simulink model "Simulacion_con_vd_export"  (R2023b)
settings: Solver=VariableStepAuto  StartTime=0.0  StopTime=2.5  RelTol=1e-3
undefined symbols (not defined in the file): alpha_cu, b_eq, C_ts, id0, J_eq, k_l, L_d, L_ls, L_q, lambda_m, magnitude, P_p, r, R_sREF, R_ts_amb, T_amb, T_sREF
libraries: SignalEditorBlockLib x7
(part 1 of 2)
settings Model: Creator=tomas  LastModifiedBy=tomas

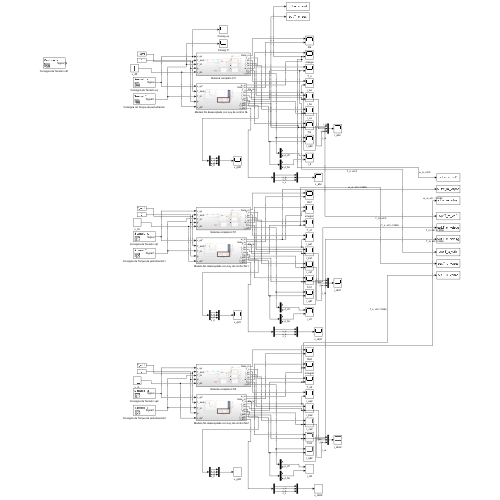
[thumbnail: Simulink's stored preview of the top-level diagram]
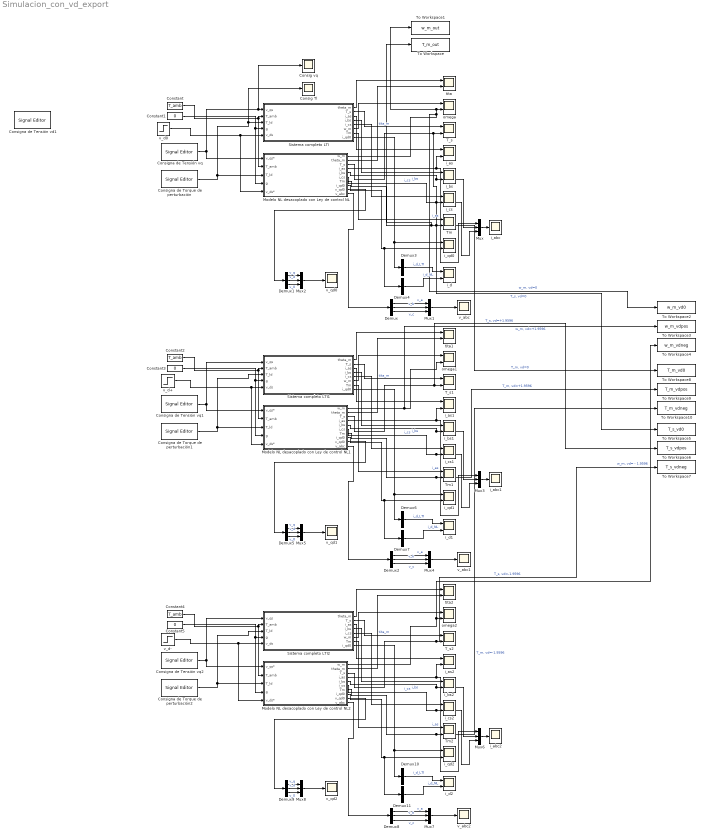
== system Simulacion_con_vd_export ==
  Consig Tl : Scope
  Consig vq : Scope
  Consigna de Tensión vd1 : SignalEditorBlockLib/Signal Editor  FileName=D:\Facu\Final AyME\Final-AyME\Simulink_LA\Simulacion\Señales\senial_vd.mat  ActiveScenario=Scenario_vd  ActiveSignal=Signal  IsBus=off  OutputBusObjectStr=Bus: BusObject  SampleTime=0  Interpolate=off  ZeroCross=off  OutputAfterFinalValue=Setting to zero  Unit=inherit  PreserveSignalName=on  ApplySigPropsToAllScenarios=on  ApplySigPropsToAllSignals=off
  Consigna de Tensión vq : SignalEditorBlockLib/Signal Editor  FileName=D:\Facu\Final AyME\Final-AyME\Simulink_LA\Simulacion\Señales\senial_vq.mat  ActiveScenario=Scenario_vq  ActiveSignal=Signal  IsBus=off  OutputBusObjectStr=Bus: BusObject  SampleTime=0  Interpolate=off  ZeroCross=off  OutputAfterFinalValue=Setting to zero  Unit=inherit  PreserveSignalName=on  ApplySigPropsToAllScenarios=on  ApplySigPropsToAllSignals=off
  Consigna de Tensión vq1 : SignalEditorBlockLib/Signal Editor  FileName=D:\Facu\Final AyME\Final-AyME\Simulink_LA\Simulacion\Señales\senial_vq.mat  ActiveScenario=Scenario_vq  ActiveSignal=Signal  IsBus=off  OutputBusObjectStr=Bus: BusObject  SampleTime=0  Interpolate=off  ZeroCross=off  OutputAfterFinalValue=Setting to zero  Unit=inherit  PreserveSignalName=on  ApplySigPropsToAllScenarios=on  ApplySigPropsToAllSignals=off
  Consigna de Tensión vq2 : SignalEditorBlockLib/Signal Editor  FileName=D:\Facu\Final AyME\Final-AyME\Simulink_LA\Simulacion\Señales\senial_vq.mat  ActiveScenario=Scenario_vq  ActiveSignal=Signal  IsBus=off  OutputBusObjectStr=Bus: BusObject  SampleTime=0  Interpolate=off  ZeroCross=off  OutputAfterFinalValue=Setting to zero  Unit=inherit  PreserveSignalName=on  ApplySigPropsToAllScenarios=on  ApplySigPropsToAllSignals=off
  Consigna de Torque de perturbación : SignalEditorBlockLib/Signal Editor  FileName=D:\Facu\Final AyME\Final-AyME\Simulink_LA\Simulacion\Señales\Signal_Tl.mat  ActiveScenario=ScenarioTl  ActiveSignal=Signal1  IsBus=off  OutputBusObjectStr=Bus: BusObject  SampleTime=0  Interpolate=off  ZeroCross=off  OutputAfterFinalValue=Setting to zero  Unit=inherit  PreserveSignalName=on  ApplySigPropsToAllScenarios=on  ApplySigPropsToAllSignals=off
  Consigna de Torque de perturbación1 : SignalEditorBlockLib/Signal Editor  FileName=D:\Facu\Final AyME\Final-AyME\Simulink_LA\Simulacion\Señales\Signal_Tl.mat  ActiveScenario=ScenarioTl  ActiveSignal=Signal1  IsBus=off  OutputBusObjectStr=Bus: BusObject  SampleTime=0  Interpolate=off  ZeroCross=off  OutputAfterFinalValue=Setting to zero  Unit=inherit  PreserveSignalName=on  ApplySigPropsToAllScenarios=on  ApplySigPropsToAllSignals=off
  Consigna de Torque de perturbación2 : SignalEditorBlockLib/Signal Editor  FileName=D:\Facu\Final AyME\Final-AyME\Simulink_LA\Simulacion\Señales\Signal_Tl.mat  ActiveScenario=ScenarioTl  ActiveSignal=Signal1  IsBus=off  OutputBusObjectStr=Bus: BusObject  SampleTime=0  Interpolate=off  ZeroCross=off  OutputAfterFinalValue=Setting to zero  Unit=inherit  PreserveSignalName=on  ApplySigPropsToAllScenarios=on  ApplySigPropsToAllSignals=off
  Constant : Constant  Value=T_amb
  Constant1 : Constant  Value=0
  Constant2 : Constant  Value=T_amb
  Constant3 : Constant  Value=0
  Constant4 : Constant  Value=T_amb
  Constant5 : Constant  Value=0
  Demux{,1..11} (12 alike) : Demux  Outputs=3
  Modelo NL desacoplado con Ley de control NL : Subsystem
  Modelo NL desacoplado con Ley de control NL1 : Subsystem
  Modelo NL desacoplado con Ley de control NL2 : Subsystem
  Mux{,1..8} (9 alike) : Mux  Inputs=3
  Sistema completo LTI : Subsystem
  Sistema completo LTI1 : Subsystem
  Sistema completo LTI2 : Subsystem
  T_s : Scope  NumInputPorts=2
  T_s1 : Scope  NumInputPorts=2
  T_s2 : Scope  NumInputPorts=2
  Tm : Scope  NumInputPorts=2
  Tm1 : Scope  NumInputPorts=2
  Tm2 : Scope  NumInputPorts=2
  To Workspace : ToWorkspace  VariableName=T_m_out  SampleTime=-1
  To Workspace1 : ToWorkspace  VariableName=w_m_out  SampleTime=-1
  To Workspace10 : ToWorkspace  VariableName=T_m_vdneg  SaveFormat=Structure With Time  SampleTime=-1
  To Workspace2 : ToWorkspace  VariableName=w_m_vd0  SaveFormat=Structure With Time  SampleTime=-1
  To Workspace3 : ToWorkspace  VariableName=w_m_vdpos  SaveFormat=Structure With Time  SampleTime=-1
  To Workspace4 : ToWorkspace  VariableName=w_m_vdneg  SaveFormat=Structure With Time  SampleTime=-1
  To Workspace5 : ToWorkspace  VariableName=T_s_vd0  SaveFormat=Structure With Time  SampleTime=-1
  To Workspace6 : ToWorkspace  VariableName=T_s_vdpos  SaveFormat=Structure With Time  SampleTime=-1
  To Workspace7 : ToWorkspace  VariableName=T_s_vdneg  SaveFormat=Structure With Time  SampleTime=-1
  To Workspace8 : ToWorkspace  VariableName=T_m_vd0  SaveFormat=Structure With Time  SampleTime=-1
  To Workspace9 : ToWorkspace  VariableName=T_m_vdpos  SaveFormat=Structure With Time  SampleTime=-1
  i_abc : Scope
  i_abc1 : Scope
  i_abc2 : Scope
  i_as : Scope  NumInputPorts=2
  i_as1 : Scope  NumInputPorts=2
  i_as2 : Scope  NumInputPorts=2
  i_bs : Scope  NumInputPorts=2
  i_bs1 : Scope  NumInputPorts=2
  i_bs2 : Scope  NumInputPorts=2
  i_cs : Scope  NumInputPorts=2
  i_cs1 : Scope  NumInputPorts=2
  i_cs2 : Scope  NumInputPorts=2
  i_d : Scope  NumInputPorts=2
  i_d1 : Scope  NumInputPorts=2
  i_d2 : Scope  NumInputPorts=2
  i_qd0 : Scope  NumInputPorts=2
  i_qd1 : Scope  NumInputPorts=2
  i_qd2 : Scope  NumInputPorts=2
  omega : Scope  NumInputPorts=2
  omega1 : Scope  NumInputPorts=2
  omega2 : Scope  NumInputPorts=2
  tita : Scope  NumInputPorts=2
  tita1 : Scope  NumInputPorts=2
  tita2 : Scope  NumInputPorts=2
  v_abc : Scope
  v_abc1 : Scope
  v_abc2 : Scope
  v_d+ : Step  Time=0.5  After=1.9596  SampleTime=0
  v_d- : Step  Time=0.5  After=-1.9596  SampleTime=0
  v_d0 : Step  Time=0  After=0  SampleTime=0
  v_qd0 : Scope
  v_qd1 : Scope
  v_qd2 : Scope
  wires:
  Demux/3 -> Mux1/3  "v_c"
  Demux1/3 -> Mux2/3  "v_0"
  Mux/1 -> i_abc/1
  Demux1/1 -> Mux2/1  "v_q"
  Mux2/1 -> v_qd0/1
  Demux1/2 -> Mux2/2  "v_d"
  Mux1/1 -> v_abc/1
  Demux/2 -> Mux1/2  "v_b"
  Demux4/2 -> i_d/2  "i_d_NL"
  Sistema completo LTI/7(Tm) -> Tm/1
  Demux/1 -> Mux1/1  "v_a"
  Sistema completo LTI/5(i_cs) -> i_cs/1
  Modelo NL desacoplado con Ley de control NL/2(theta_m) -> tita/2  "tita_m"
  Sistema completo LTI/1(theta_m) -> tita/1
  Demux3/2 -> i_d/1  "i_d_LTI"
  Sistema completo LTI/3(i_as) -> i_as/1
  Constant/1 -> Modelo NL desacoplado con Ley de control NL/2(T_amb), Sistema completo LTI/2(T_amb)
  Modelo NL desacoplado con Ley de control NL/9(v_qd0) -> Demux1/1
  Consigna de Torque de perturbación/1 -> Modelo NL desacoplado con Ley de control NL/3(T_ld), Consig Tl/1, Sistema completo LTI/3(T_ld)
  Modelo NL desacoplado con Ley de control NL/4(i_as) -> Mux/1, i_as/2  "i_as"
  Modelo NL desacoplado con Ley de control NL/6(i_cs) -> i_cs/2, Mux/3  "i_cs"
  Constant1/1 -> Modelo NL desacoplado con Ley de control NL/4(g), Sistema completo LTI/4(g)
  Sistema completo LTI/4(i_bs) -> i_bs/1
  Modelo NL desacoplado con Ley de control NL/7(Tm) -> To Workspace8/1, Tm/2, To Workspace/1  "T_m, vd=0"
  Sistema completo LTI/8(i_qd0) -> Demux3/1, i_qd0/1
  Modelo NL desacoplado con Ley de control NL/8(i_qd0) -> i_qd0/2, Demux4/1
  Modelo NL desacoplado con Ley de control NL/10(v_abc) -> Demux/1
  Sistema completo LTI/6(w_m) -> omega/1
  Consigna de Tensión vq/1 -> Consig vq/1, Sistema completo LTI/1(v_qs), Modelo NL desacoplado con Ley de control NL/1(v_qs*)
  Sistema completo LTI/2(T_s) -> T_s/1
  Modelo NL desacoplado con Ley de control NL/5(i_bs) -> Mux/2, i_bs/2  "i_bs"
  v_d0/1 -> Modelo NL desacoplado con Ley de control NL/5(v_ds*), Sistema completo LTI/5(v_ds)
  Modelo NL desacoplado con Ley de control NL1/5(i_bs) -> Mux3/2, i_bs1/2  "i_bs"
  Modelo NL desacoplado con Ley de control NL1/10(v_abc) -> Demux2/1
  Sistema completo LTI1/6(w_m) -> omega1/1
  Modelo NL desacoplado con Ley de control NL1/6(i_cs) -> i_cs1/2, Mux3/3  "i_cs"
  Constant3/1 -> Modelo NL desacoplado con Ley de control NL1/4(g), Sistema completo LTI1/4(g)
  Modelo NL desacoplado con Ley de control NL1/4(i_as) -> Mux3/1, i_as1/2  "i_as"
  Consigna de Torque de perturbación1/1 -> Modelo NL desacoplado con Ley de control NL1/3(T_ld), Sistema completo LTI1/3(T_ld)
  Sistema completo LTI1/4(i_bs) -> i_bs1/1
  Modelo NL desacoplado con Ley de control NL1/3(T_s) -> To Workspace6/1, T_s1/2  "T_s, vd=+1.9596"
  Modelo NL desacoplado con Ley de control NL1/9(v_qd0) -> Demux5/1
  Demux6/2 -> i_d1/1  "i_d_LTI"
  Consigna de Tensión vq1/1 -> Sistema completo LTI1/1(v_qs), Modelo NL desacoplado con Ley de control NL1/1(v_qs*)
  Sistema completo LTI1/1(theta_m) -> tita1/1
  Constant2/1 -> Modelo NL desacoplado con Ley de control NL1/2(T_amb), Sistema completo LTI1/2(T_amb)
  Sistema completo LTI1/2(T_s) -> T_s1/1
  Sistema completo LTI1/7(Tm) -> Tm1/1
  Demux2/1 -> Mux4/1  "v_a"
  Demux7/2 -> i_d1/2  "i_d_NL"
  Demux2/2 -> Mux4/2  "v_b"
  Sistema completo LTI1/5(i_cs) -> i_cs1/1
  Mux3/1 -> i_abc1/1
  Demux2/3 -> Mux4/3  "v_c"
  Demux5/3 -> Mux5/3  "v_0"
  Sistema completo LTI1/3(i_as) -> i_as1/1
  Modelo NL desacoplado con Ley de control NL1/7(Tm) -> To Workspace9/1, Tm1/2  "T_m, vd=+1.9596"
  Mux4/1 -> v_abc1/1
  v_d+/1 -> Sistema completo LTI1/5(v_ds), Modelo NL desacoplado con Ley de control NL1/5(v_ds*)
  Demux5/1 -> Mux5/1  "v_q"
  Modelo NL desacoplado con Ley de control NL1/8(i_qd0) -> i_qd1/2, Demux7/1
  Demux5/2 -> Mux5/2  "v_d"
  Modelo NL desacoplado con Ley de control NL1/2(theta_m) -> tita1/2  "tita_m"
  Sistema completo LTI1/8(i_qd0) -> Demux6/1, i_qd1/1
  Mux5/1 -> v_qd1/1
  Demux11/2 -> i_d2/2  "i_d_NL"
  Demux8/1 -> Mux7/1  "v_a"
  Modelo NL desacoplado con Ley de control NL2/1(w_m) -> To Workspace4/1, omega2/2  "w_m, vd= - 1.9596"
  Sistema completo LTI2/1(theta_m) -> tita2/1
  Consigna de Tensión vq2/1 -> Sistema completo LTI2/1(v_qs), Modelo NL desacoplado con Ley de control NL2/1(v_qs*)
  Constant4/1 -> Modelo NL desacoplado con Ley de control NL2/2(T_amb), Sistema completo LTI2/2(T_amb)
  Sistema completo LTI2/7(Tm) -> Tm2/1
  Consigna de Torque de perturbación2/1 -> Modelo NL desacoplado con Ley de control NL2/3(T_ld), Sistema completo LTI2/3(T_ld)
  Modelo NL desacoplado con Ley de control NL2/9(v_qd0) -> Demux9/1
  Modelo NL desacoplado con Ley de control NL2/3(T_s) -> To Workspace7/1, T_s2/2  "T_s, vd=-1.9596"
  Modelo NL desacoplado con Ley de control NL2/6(i_cs) -> i_cs2/2, Mux6/3  "i_cs"
  Modelo NL desacoplado con Ley de control NL2/5(i_bs) -> Mux6/2, i_bs2/2  "i_bs"
  Constant5/1 -> Modelo NL desacoplado con Ley de control NL2/4(g), Sistema completo LTI2/4(g)
  Modelo NL desacoplado con Ley de control NL2/10(v_abc) -> Demux8/1
  Demux10/2 -> i_d2/1  "i_d_LTI"
  Sistema completo LTI2/4(i_bs) -> i_bs2/1
  Demux8/2 -> Mux7/2  "v_b"
  Sistema completo LTI2/6(w_m) -> omega2/1
  Sistema completo LTI2/2(T_s) -> T_s2/1
  Mux8/1 -> v_qd2/1
  Modelo NL desacoplado con Ley de control NL2/2(theta_m) -> tita2/2  "tita_m"
  Sistema completo LTI2/8(i_qd0) -> Demux10/1, i_qd2/1
  Demux9/2 -> Mux8/2  "v_d"
  Modelo NL desacoplado con Ley de control NL2/8(i_qd0) -> i_qd2/2, Demux11/1
  Demux9/1 -> Mux8/1  "v_q"
  Modelo NL desacoplado con Ley de control NL2/4(i_as) -> Mux6/1, i_as2/2  "i_as"
  Mux7/1 -> v_abc2/1
  Demux8/3 -> Mux7/3  "v_c"
  Sistema completo LTI2/3(i_as) -> i_as2/1
  Demux9/3 -> Mux8/3  "v_0"
  Mux6/1 -> i_abc2/1
  v_d-/1 -> Modelo NL desacoplado con Ley de control NL2/5(v_ds*), Sistema completo LTI2/5(v_ds)
  Sistema completo LTI2/5(i_cs) -> i_cs2/1
  Modelo NL desacoplado con Ley de control NL1/1(w_m) -> To Workspace3/1, omega1/2  "w_m, vd=+1.9596"
  Modelo NL desacoplado con Ley de control NL/1(w_m) -> To Workspace2/1, To Workspace1/1, omega/2  "w_m, vd=0"
  Modelo NL desacoplado con Ley de control NL2/7(Tm) -> To Workspace10/1, Tm2/2  "T_m, vd=-1.9596"
  Modelo NL desacoplado con Ley de control NL/3(T_s) -> To Workspace5/1, T_s/2  "T_s, vd=0"

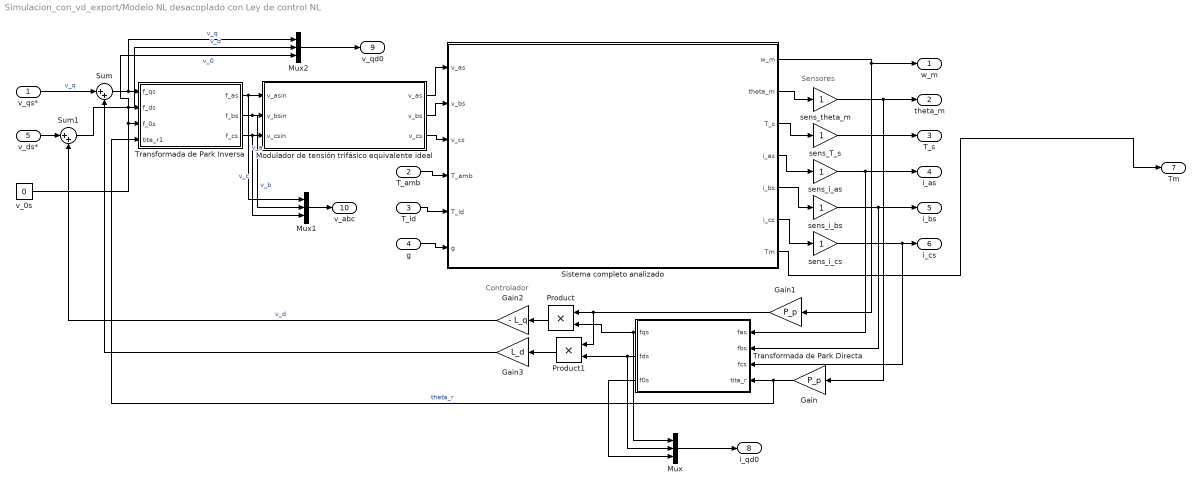
== system Simulacion_con_vd_export/Modelo NL desacoplado con Ley de control NL ==
  note: Sensores
  note: Controlador
  v_qs* : Inport
  T_amb : Inport  Port=2
  T_ld : Inport  Port=3
  g : Inport  Port=4
  v_ds* : Inport  Port=5
  Gain : Gain  Gain=P_p
  Gain1 : Gain  Gain=P_p
  Gain2 : Gain  Gain=- L_q
  Gain3 : Gain  Gain=L_d
  Modulador de tensión trifásico equivalente ideal : MATLAB Function  TreatAsAtomicUnit=on
  Mux : Mux  Inputs=3
  Mux1 : Mux  Inputs=3
  Mux2 : Mux  Inputs=3
  Product : Product
  Product1 : Product
  "Sistema completo analizado " : Subsystem
  Sum : Sum  Inputs=|++
  Sum1 : Sum  Inputs=|++
  Transformada de Park Directa : Subsystem
  Transformada de Park Inversa : Subsystem
  sens_T_s : Gain
  sens_i_as : Gain
  sens_i_bs : Gain
  sens_i_cs : Gain
  sens_theta_m : Gain
  v_0s : Constant  Value=0
  w_m : Outport
  theta_m : Outport  Port=2
  T_s : Outport  Port=3
  i_as : Outport  Port=4
  i_bs : Outport  Port=5
  i_cs : Outport  Port=6
  Tm : Outport  Port=7
  i_qd0 : Outport  Port=8
  v_qd0 : Outport  Port=9
  v_abc : Outport  Port=10
  wires:
  "Sistema completo analizado "/5(i_bs) -> sens_i_bs/1
  Gain1/1 -> Product1/1, Product/1
  Transformada de Park Directa/3(f0s) -> Mux/3
  T_amb/1 -> "Sistema completo analizado "/4(T_amb)
  "Sistema completo analizado "/3(T_s) -> sens_T_s/1
  g/1 -> "Sistema completo analizado "/6(g)
  Modulador de tensión trifásico equivalente ideal/2(v_bs) -> "Sistema completo analizado "/2(v_bs)
  sens_T_s/1 -> T_s/1
  Transformada de Park Directa/1(fqs) -> Mux/1, Product/2
  Modulador de tensión trifásico equivalente ideal/1(v_as) -> "Sistema completo analizado "/1(v_as)
  sens_i_as/1 -> Transformada de Park Directa/1(fas), i_as/1
  "Sistema completo analizado "/6(i_cs) -> sens_i_cs/1
  "Sistema completo analizado "/4(i_as) -> sens_i_as/1
  Transformada de Park Inversa/3(f_cs) -> Mux1/3, Modulador de tensión trifásico equivalente ideal/3(v_csin)  "v_c"
  Transformada de Park Inversa/1(f_as) -> Mux1/1, Modulador de tensión trifásico equivalente ideal/1(v_asin)  "v_a"
  Transformada de Park Inversa/2(f_bs) -> Mux1/2, Modulador de tensión trifásico equivalente ideal/2(v_bsin)  "v_b"
  Product1/1 -> Gain3/1
  "Sistema completo analizado "/2(theta_m) -> sens_theta_m/1
  Transformada de Park Directa/2(fds) -> Mux/2, Product1/2
  sens_theta_m/1 -> Gain/1, theta_m/1
  sens_i_bs/1 -> Transformada de Park Directa/2(fbs), i_bs/1
  v_0s/1 -> Mux2/3, Transformada de Park Inversa/3(f_0s)  "v_0"
  Gain/1 -> Transformada de Park Inversa/4(tita_r1), Transformada de Park Directa/4(tita_r)  "theta_r"
  Gain2/1 -> Sum1/2  "v_d"
  Product/1 -> Gain2/1
  Modulador de tensión trifásico equivalente ideal/3(v_cs) -> "Sistema completo analizado "/3(v_cs)
  Sum/1 -> Mux2/1, Transformada de Park Inversa/1(f_qs)  "v_q"
  sens_i_cs/1 -> Transformada de Park Directa/3(fcs), i_cs/1
  T_ld/1 -> "Sistema completo analizado "/5(T_ld)
  Gain3/1 -> Sum/2
  "Sistema completo analizado "/1(w_m) -> Gain1/1, w_m/1
  "Sistema completo analizado "/7(Tm) -> Tm/1
  Mux/1 -> i_qd0/1
  Mux1/1 -> v_abc/1
  Mux2/1 -> v_qd0/1
  Sum1/1 -> Mux2/2, Transformada de Park Inversa/2(f_ds)  "v_d"
  v_ds*/1 -> Sum1/1
  v_qs*/1 -> Sum/1  "v_q"

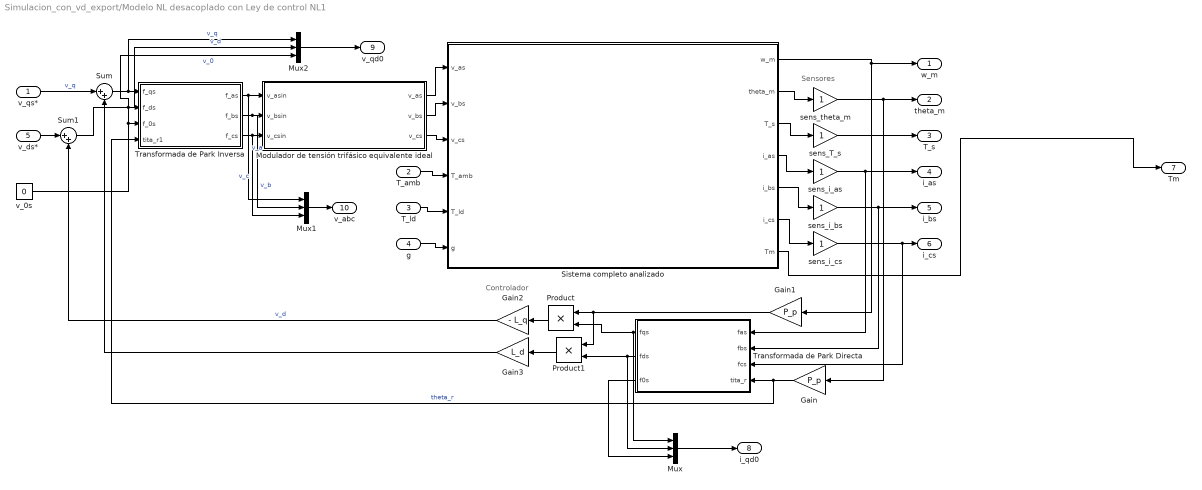
== system Simulacion_con_vd_export/Modelo NL desacoplado con Ley de control NL1 ==
  note: Sensores
  note: Controlador
  v_qs* : Inport
  T_amb : Inport  Port=2
  T_ld : Inport  Port=3
  g : Inport  Port=4
  v_ds* : Inport  Port=5
  Gain : Gain  Gain=P_p
  Gain1 : Gain  Gain=P_p
  Gain2 : Gain  Gain=- L_q
  Gain3 : Gain  Gain=L_d
  Modulador de tensión trifásico equivalente ideal : MATLAB Function  TreatAsAtomicUnit=on
  Mux : Mux  Inputs=3
  Mux1 : Mux  Inputs=3
  Mux2 : Mux  Inputs=3
  Product : Product
  Product1 : Product
  "Sistema completo analizado " : Subsystem
  Sum : Sum  Inputs=|++
  Sum1 : Sum  Inputs=|++
  Transformada de Park Directa : Subsystem
  Transformada de Park Inversa : Subsystem
  sens_T_s : Gain
  sens_i_as : Gain
  sens_i_bs : Gain
  sens_i_cs : Gain
  sens_theta_m : Gain
  v_0s : Constant  Value=0
  w_m : Outport
  theta_m : Outport  Port=2
  T_s : Outport  Port=3
  i_as : Outport  Port=4
  i_bs : Outport  Port=5
  i_cs : Outport  Port=6
  Tm : Outport  Port=7
  i_qd0 : Outport  Port=8
  v_qd0 : Outport  Port=9
  v_abc : Outport  Port=10
  wires:
  "Sistema completo analizado "/5(i_bs) -> sens_i_bs/1
  Gain1/1 -> Product1/1, Product/1
  Transformada de Park Directa/3(f0s) -> Mux/3
  T_amb/1 -> "Sistema completo analizado "/4(T_amb)
  "Sistema completo analizado "/3(T_s) -> sens_T_s/1
  g/1 -> "Sistema completo analizado "/6(g)
  Modulador de tensión trifásico equivalente ideal/2(v_bs) -> "Sistema completo analizado "/2(v_bs)
  sens_T_s/1 -> T_s/1
  Transformada de Park Directa/1(fqs) -> Mux/1, Product/2
  Modulador de tensión trifásico equivalente ideal/1(v_as) -> "Sistema completo analizado "/1(v_as)
  sens_i_as/1 -> Transformada de Park Directa/1(fas), i_as/1
  "Sistema completo analizado "/6(i_cs) -> sens_i_cs/1
  "Sistema completo analizado "/4(i_as) -> sens_i_as/1
  Transformada de Park Inversa/3(f_cs) -> Mux1/3, Modulador de tensión trifásico equivalente ideal/3(v_csin)  "v_c"
  Transformada de Park Inversa/1(f_as) -> Mux1/1, Modulador de tensión trifásico equivalente ideal/1(v_asin)  "v_a"
  Transformada de Park Inversa/2(f_bs) -> Mux1/2, Modulador de tensión trifásico equivalente ideal/2(v_bsin)  "v_b"
  Product1/1 -> Gain3/1
  "Sistema completo analizado "/2(theta_m) -> sens_theta_m/1
  Transformada de Park Directa/2(fds) -> Mux/2, Product1/2
  sens_theta_m/1 -> Gain/1, theta_m/1
  sens_i_bs/1 -> Transformada de Park Directa/2(fbs), i_bs/1
  v_0s/1 -> Mux2/3, Transformada de Park Inversa/3(f_0s)  "v_0"
  Gain/1 -> Transformada de Park Inversa/4(tita_r1), Transformada de Park Directa/4(tita_r)  "theta_r"
  Gain2/1 -> Sum1/2  "v_d"
  Product/1 -> Gain2/1
  Modulador de tensión trifásico equivalente ideal/3(v_cs) -> "Sistema completo analizado "/3(v_cs)
  Sum/1 -> Mux2/1, Transformada de Park Inversa/1(f_qs)  "v_q"
  sens_i_cs/1 -> Transformada de Park Directa/3(fcs), i_cs/1
  T_ld/1 -> "Sistema completo analizado "/5(T_ld)
  Gain3/1 -> Sum/2
  "Sistema completo analizado "/1(w_m) -> Gain1/1, w_m/1
  "Sistema completo analizado "/7(Tm) -> Tm/1
  Mux/1 -> i_qd0/1
  Mux1/1 -> v_abc/1
  Mux2/1 -> v_qd0/1
  Sum1/1 -> Mux2/2, Transformada de Park Inversa/2(f_ds)  "v_d"
  v_ds*/1 -> Sum1/1
  v_qs*/1 -> Sum/1  "v_q"

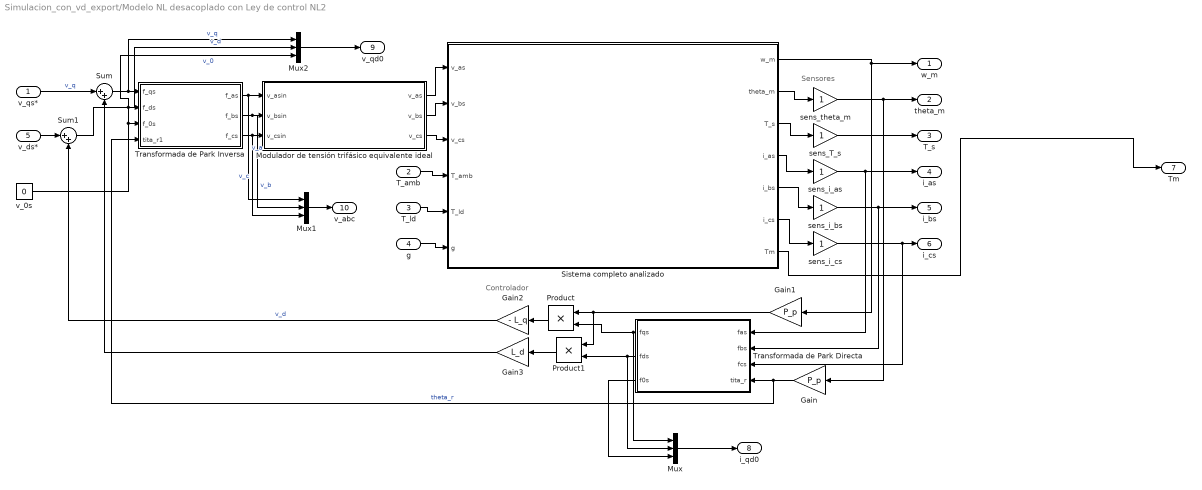
== system Simulacion_con_vd_export/Modelo NL desacoplado con Ley de control NL2 ==
  note: Sensores
  note: Controlador
  v_qs* : Inport
  T_amb : Inport  Port=2
  T_ld : Inport  Port=3
  g : Inport  Port=4
  v_ds* : Inport  Port=5
  Gain : Gain  Gain=P_p
  Gain1 : Gain  Gain=P_p
  Gain2 : Gain  Gain=- L_q
  Gain3 : Gain  Gain=L_d
  Modulador de tensión trifásico equivalente ideal : MATLAB Function  TreatAsAtomicUnit=on
  Mux : Mux  Inputs=3
  Mux1 : Mux  Inputs=3
  Mux2 : Mux  Inputs=3
  Product : Product
  Product1 : Product
  "Sistema completo analizado " : Subsystem
  Sum : Sum  Inputs=|++
  Sum1 : Sum  Inputs=|++
  Transformada de Park Directa : Subsystem
  Transformada de Park Inversa : Subsystem
  sens_T_s : Gain
  sens_i_as : Gain
  sens_i_bs : Gain
  sens_i_cs : Gain
  sens_theta_m : Gain
  v_0s : Constant  Value=0
  w_m : Outport
  theta_m : Outport  Port=2
  T_s : Outport  Port=3
  i_as : Outport  Port=4
  i_bs : Outport  Port=5
  i_cs : Outport  Port=6
  Tm : Outport  Port=7
  i_qd0 : Outport  Port=8
  v_qd0 : Outport  Port=9
  v_abc : Outport  Port=10
  wires:
  "Sistema completo analizado "/5(i_bs) -> sens_i_bs/1
  Gain1/1 -> Product1/1, Product/1
  Transformada de Park Directa/3(f0s) -> Mux/3
  T_amb/1 -> "Sistema completo analizado "/4(T_amb)
  "Sistema completo analizado "/3(T_s) -> sens_T_s/1
  g/1 -> "Sistema completo analizado "/6(g)
  Modulador de tensión trifásico equivalente ideal/2(v_bs) -> "Sistema completo analizado "/2(v_bs)
  sens_T_s/1 -> T_s/1
  Transformada de Park Directa/1(fqs) -> Mux/1, Product/2
  Modulador de tensión trifásico equivalente ideal/1(v_as) -> "Sistema completo analizado "/1(v_as)
  sens_i_as/1 -> Transformada de Park Directa/1(fas), i_as/1
  "Sistema completo analizado "/6(i_cs) -> sens_i_cs/1
  "Sistema completo analizado "/4(i_as) -> sens_i_as/1
  Transformada de Park Inversa/3(f_cs) -> Mux1/3, Modulador de tensión trifásico equivalente ideal/3(v_csin)  "v_c"
  Transformada de Park Inversa/1(f_as) -> Mux1/1, Modulador de tensión trifásico equivalente ideal/1(v_asin)  "v_a"
  Transformada de Park Inversa/2(f_bs) -> Mux1/2, Modulador de tensión trifásico equivalente ideal/2(v_bsin)  "v_b"
  Product1/1 -> Gain3/1
  "Sistema completo analizado "/2(theta_m) -> sens_theta_m/1
  Transformada de Park Directa/2(fds) -> Mux/2, Product1/2
  sens_theta_m/1 -> Gain/1, theta_m/1
  sens_i_bs/1 -> Transformada de Park Directa/2(fbs), i_bs/1
  v_0s/1 -> Mux2/3, Transformada de Park Inversa/3(f_0s)  "v_0"
  Gain/1 -> Transformada de Park Inversa/4(tita_r1), Transformada de Park Directa/4(tita_r)  "theta_r"
  Gain2/1 -> Sum1/2  "v_d"
  Product/1 -> Gain2/1
  Modulador de tensión trifásico equivalente ideal/3(v_cs) -> "Sistema completo analizado "/3(v_cs)
  Sum/1 -> Mux2/1, Transformada de Park Inversa/1(f_qs)  "v_q"
  sens_i_cs/1 -> Transformada de Park Directa/3(fcs), i_cs/1
  T_ld/1 -> "Sistema completo analizado "/5(T_ld)
  Gain3/1 -> Sum/2
  "Sistema completo analizado "/1(w_m) -> Gain1/1, w_m/1
  "Sistema completo analizado "/7(Tm) -> Tm/1
  Mux/1 -> i_qd0/1
  Mux1/1 -> v_abc/1
  Mux2/1 -> v_qd0/1
  Sum1/1 -> Mux2/2, Transformada de Park Inversa/2(f_ds)  "v_d"
  v_ds*/1 -> Sum1/1
  v_qs*/1 -> Sum/1  "v_q"

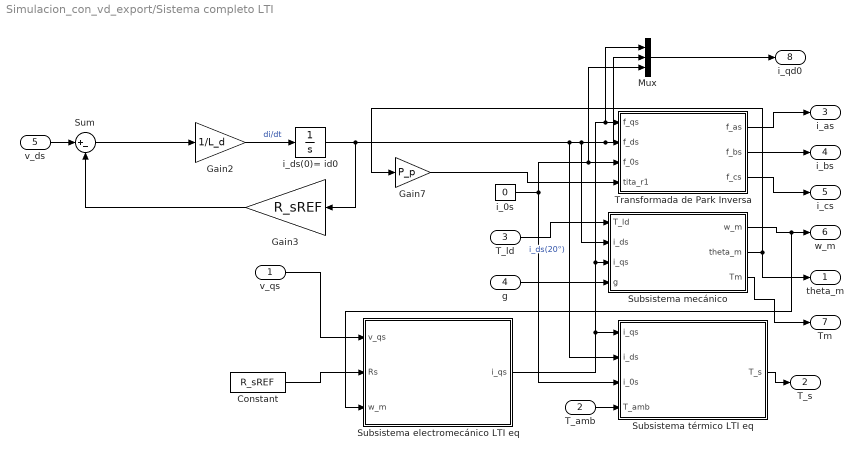
== system Simulacion_con_vd_export/Sistema completo LTI ==
  v_qs : Inport
  T_amb : Inport  Port=2
  T_ld : Inport  Port=3
  g : Inport  Port=4
  v_ds : Inport  Port=5
  Constant : Constant  Value=R_sREF
  Gain2 : Gain  Gain=1/L_d
  Gain3 : Gain  Gain=R_sREF
  Gain7 : Gain  Gain=P_p
  Mux : Mux  Inputs=3
  Subsistema electromecánico LTI eq : Subsystem
  Subsistema mecánico : Subsystem
  Subsistema térmico LTI eq : Subsystem
  Sum : Sum  Inputs=|+-
  Transformada de Park Inversa : Subsystem
  i_0s : Constant  Value=0
  i_ds(0)= id0 : Integrator  InitialCondition=id0
  theta_m : Outport
  T_s : Outport  Port=2
  i_as : Outport  Port=3
  i_bs : Outport  Port=4
  i_cs : Outport  Port=5
  w_m : Outport  Port=6
  Tm : Outport  Port=7
  i_qd0 : Outport  Port=8
  wires:
  Subsistema mecánico/2(theta_m) -> theta_m/1, Gain7/1
  v_qs/1 -> Subsistema electromecánico LTI eq/1(v_qs)
  Transformada de Park Inversa/1(f_as) -> i_as/1
  T_ld/1 -> Subsistema mecánico/1(T_ld)
  Transformada de Park Inversa/2(f_bs) -> i_bs/1
  Subsistema térmico LTI eq/1(T_s) -> T_s/1
  Transformada de Park Inversa/3(f_cs) -> i_cs/1
  Subsistema mecánico/1(w_m) -> Subsistema electromecánico LTI eq/3(w_m), w_m/1
  T_amb/1 -> Subsistema térmico LTI eq/4(T_amb)
  i_0s/1 -> Subsistema térmico LTI eq/3(i_0s), Transformada de Park Inversa/3(f_0s), Mux/3
  Subsistema electromecánico LTI eq/1(i_qs) -> Subsistema mecánico/3(i_qs), Mux/1, Transformada de Park Inversa/1(f_qs), Subsistema térmico LTI eq/1(i_qs)
  Gain7/1 -> Transformada de Park Inversa/4(tita_r1)
  i_ds(0)= id0/1 -> Subsistema mecánico/2(i_ds), Mux/2, Transformada de Park Inversa/2(f_ds), Subsistema térmico LTI eq/2(i_ds), Gain3/1  "i_ds(20°)"
  Gain2/1 -> i_ds(0)= id0/1  "di/dt"
  g/1 -> Subsistema mecánico/4(g)
  Subsistema mecánico/3(Tm) -> Tm/1
  Mux/1 -> i_qd0/1
  Constant/1 -> Subsistema electromecánico LTI eq/2(Rs)
  Gain3/1 -> Sum/2
  v_ds/1 -> Sum/1
  Sum/1 -> Gain2/1

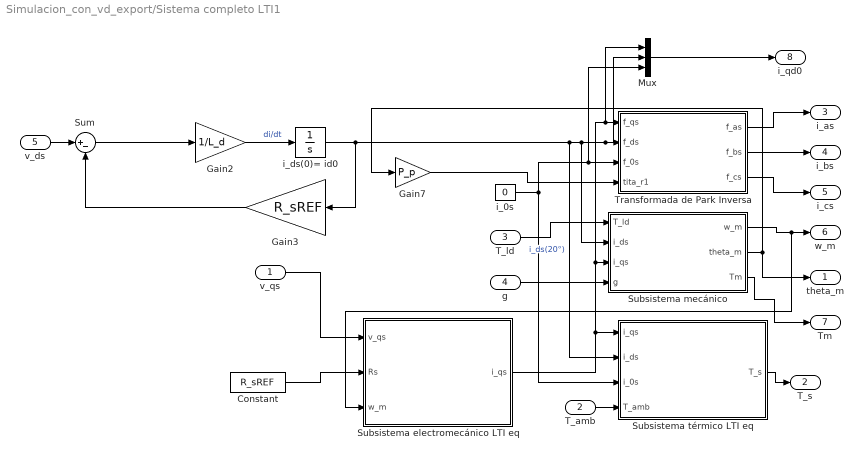
== system Simulacion_con_vd_export/Sistema completo LTI1 ==
  v_qs : Inport
  T_amb : Inport  Port=2
  T_ld : Inport  Port=3
  g : Inport  Port=4
  v_ds : Inport  Port=5
  Constant : Constant  Value=R_sREF
  Gain2 : Gain  Gain=1/L_d
  Gain3 : Gain  Gain=R_sREF
  Gain7 : Gain  Gain=P_p
  Mux : Mux  Inputs=3
  Subsistema electromecánico LTI eq : Subsystem
  Subsistema mecánico : Subsystem
  Subsistema térmico LTI eq : Subsystem
  Sum : Sum  Inputs=|+-
  Transformada de Park Inversa : Subsystem
  i_0s : Constant  Value=0
  i_ds(0)= id0 : Integrator  InitialCondition=id0
  theta_m : Outport
  T_s : Outport  Port=2
  i_as : Outport  Port=3
  i_bs : Outport  Port=4
  i_cs : Outport  Port=5
  w_m : Outport  Port=6
  Tm : Outport  Port=7
  i_qd0 : Outport  Port=8
  wires:
  Subsistema mecánico/2(theta_m) -> theta_m/1, Gain7/1
  v_qs/1 -> Subsistema electromecánico LTI eq/1(v_qs)
  Transformada de Park Inversa/1(f_as) -> i_as/1
  T_ld/1 -> Subsistema mecánico/1(T_ld)
  Transformada de Park Inversa/2(f_bs) -> i_bs/1
  Subsistema térmico LTI eq/1(T_s) -> T_s/1
  Transformada de Park Inversa/3(f_cs) -> i_cs/1
  Subsistema mecánico/1(w_m) -> Subsistema electromecánico LTI eq/3(w_m), w_m/1
  T_amb/1 -> Subsistema térmico LTI eq/4(T_amb)
  i_0s/1 -> Subsistema térmico LTI eq/3(i_0s), Transformada de Park Inversa/3(f_0s), Mux/3
  Subsistema electromecánico LTI eq/1(i_qs) -> Subsistema mecánico/3(i_qs), Mux/1, Transformada de Park Inversa/1(f_qs), Subsistema térmico LTI eq/1(i_qs)
  Gain7/1 -> Transformada de Park Inversa/4(tita_r1)
  i_ds(0)= id0/1 -> Subsistema mecánico/2(i_ds), Mux/2, Transformada de Park Inversa/2(f_ds), Subsistema térmico LTI eq/2(i_ds), Gain3/1  "i_ds(20°)"
  Gain2/1 -> i_ds(0)= id0/1  "di/dt"
  g/1 -> Subsistema mecánico/4(g)
  Subsistema mecánico/3(Tm) -> Tm/1
  Mux/1 -> i_qd0/1
  Constant/1 -> Subsistema electromecánico LTI eq/2(Rs)
  Gain3/1 -> Sum/2
  v_ds/1 -> Sum/1
  Sum/1 -> Gain2/1

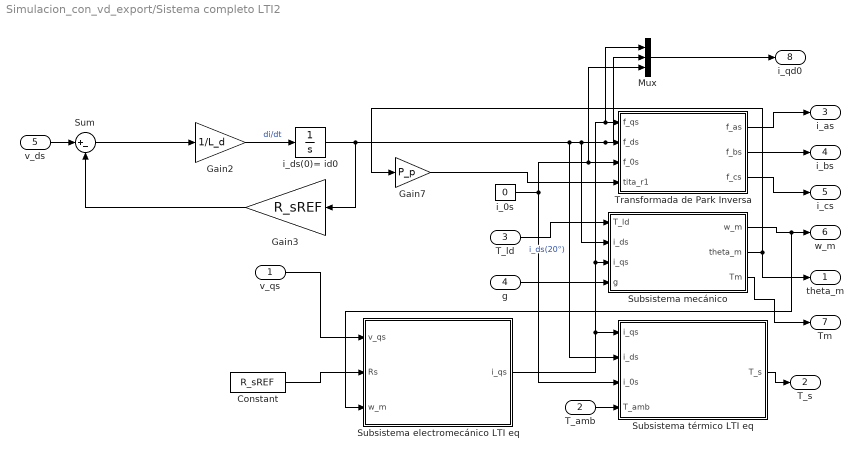
== system Simulacion_con_vd_export/Sistema completo LTI2 ==
  v_qs : Inport
  T_amb : Inport  Port=2
  T_ld : Inport  Port=3
  g : Inport  Port=4
  v_ds : Inport  Port=5
  Constant : Constant  Value=R_sREF
  Gain2 : Gain  Gain=1/L_d
  Gain3 : Gain  Gain=R_sREF
  Gain7 : Gain  Gain=P_p
  Mux : Mux  Inputs=3
  Subsistema electromecánico LTI eq : Subsystem
  Subsistema mecánico : Subsystem
  Subsistema térmico LTI eq : Subsystem
  Sum : Sum  Inputs=|+-
  Transformada de Park Inversa : Subsystem
  i_0s : Constant  Value=0
  i_ds(0)= id0 : Integrator  InitialCondition=id0
  theta_m : Outport
  T_s : Outport  Port=2
  i_as : Outport  Port=3
  i_bs : Outport  Port=4
  i_cs : Outport  Port=5
  w_m : Outport  Port=6
  Tm : Outport  Port=7
  i_qd0 : Outport  Port=8
  wires:
  Subsistema mecánico/2(theta_m) -> theta_m/1, Gain7/1
  v_qs/1 -> Subsistema electromecánico LTI eq/1(v_qs)
  Transformada de Park Inversa/1(f_as) -> i_as/1
  T_ld/1 -> Subsistema mecánico/1(T_ld)
  Transformada de Park Inversa/2(f_bs) -> i_bs/1
  Subsistema térmico LTI eq/1(T_s) -> T_s/1
  Transformada de Park Inversa/3(f_cs) -> i_cs/1
  Subsistema mecánico/1(w_m) -> Subsistema electromecánico LTI eq/3(w_m), w_m/1
  T_amb/1 -> Subsistema térmico LTI eq/4(T_amb)
  i_0s/1 -> Subsistema térmico LTI eq/3(i_0s), Transformada de Park Inversa/3(f_0s), Mux/3
  Subsistema electromecánico LTI eq/1(i_qs) -> Subsistema mecánico/3(i_qs), Mux/1, Transformada de Park Inversa/1(f_qs), Subsistema térmico LTI eq/1(i_qs)
  Gain7/1 -> Transformada de Park Inversa/4(tita_r1)
  i_ds(0)= id0/1 -> Subsistema mecánico/2(i_ds), Mux/2, Transformada de Park Inversa/2(f_ds), Subsistema térmico LTI eq/2(i_ds), Gain3/1  "i_ds(20°)"
  Gain2/1 -> i_ds(0)= id0/1  "di/dt"
  g/1 -> Subsistema mecánico/4(g)
  Subsistema mecánico/3(Tm) -> Tm/1
  Mux/1 -> i_qd0/1
  Constant/1 -> Subsistema electromecánico LTI eq/2(Rs)
  Gain3/1 -> Sum/2
  v_ds/1 -> Sum/1
  Sum/1 -> Gain2/1

== system Simulacion_con_vd_export/Modelo NL desacoplado con Ley de control NL/Sistema completo analizado  ==
  v_as : Inport
  v_bs : Inport  Port=2
  v_cs : Inport  Port=3
  T_amb : Inport  Port=4
  T_ld : Inport  Port=5
  g : Inport  Port=6
  Gain : Gain  Gain=P_p
  Subsistema electromecánico : Subsystem
  Subsistema mecánico : Subsystem
  Subsistema térmico1 : Subsystem
  To Workspace : ToWorkspace  VariableName=iq  SampleTime=-1
  Transformada de Park Directa : Subsystem
  Transformada de Park Inversa : Subsystem
  w_m : Outport
  theta_m : Outport  Port=2
  T_s : Outport  Port=3
  i_as : Outport  Port=4
  i_bs : Outport  Port=5
  i_cs : Outport  Port=6
  Tm : Outport  Port=7
  wires:
  Transformada de Park Inversa/3(f_cs) -> i_cs/1
  Subsistema mecánico/1(w_m) -> w_m/1, Subsistema electromecánico/5(w_m)
  Subsistema electromecánico/3(i_0s) -> Subsistema térmico1/3(i_0s), Transformada de Park Inversa/3(f_0s)
  Transformada de Park Directa/1(fqs) -> Subsistema electromecánico/1(v_qs)
  Subsistema térmico1/2(T_s) -> T_s/1
  Transformada de Park Directa/3(f0s) -> Subsistema electromecánico/3(v_0s)
  Subsistema electromecánico/2(i_ds) -> Subsistema térmico1/2(i_ds), Transformada de Park Inversa/2(f_ds), Subsistema mecánico/2(i_ds)
  Gain/1 -> Transformada de Park Inversa/4(tita_r1), Transformada de Park Directa/4(tita_r)
  T_ld/1 -> Subsistema mecánico/1(T_ld)
  Transformada de Park Directa/2(fds) -> Subsistema electromecánico/2(v_ds)
  Transformada de Park Inversa/2(f_bs) -> i_bs/1
  v_bs/1 -> Transformada de Park Directa/2(fbs)
  T_amb/1 -> Subsistema térmico1/4(T_amb)
  Transformada de Park Inversa/1(f_as) -> i_as/1
  v_as/1 -> Transformada de Park Directa/1(fas)
  Subsistema mecánico/2(theta_m) -> Gain/1, theta_m/1
  v_cs/1 -> Transformada de Park Directa/3(fcs)
  Subsistema electromecánico/1(i_qs) -> To Workspace/1, Transformada de Park Inversa/1(f_qs), Subsistema mecánico/3(i_qs), Subsistema térmico1/1(i_qs)
  Subsistema térmico1/1(R_s) -> Subsistema electromecánico/4(Rs)
  g/1 -> Subsistema mecánico/4(g)
  Subsistema mecánico/3(Tm) -> Tm/1

== system Simulacion_con_vd_export/Modelo NL desacoplado con Ley de control NL/Transformada de Park Directa ==
  fas : Inport
  fbs : Inport  Port=2
  fcs : Inport  Port=3
  tita_r : Inport  Port=4
  MATLAB Function1 : MATLAB Function  TreatAsAtomicUnit=on
  fqs : Outport
  fds : Outport  Port=2
  f0s : Outport  Port=3
  wires:
  fas/1 -> MATLAB Function1/1(f_as)
  MATLAB Function1/3(f_0s) -> f0s/1
  MATLAB Function1/2(f_ds) -> fds/1
  fbs/1 -> MATLAB Function1/2(f_bs)
  fcs/1 -> MATLAB Function1/3(f_cs)
  tita_r/1 -> MATLAB Function1/4(tita_r)
  MATLAB Function1/1(f_qs) -> fqs/1

== system Simulacion_con_vd_export/Modelo NL desacoplado con Ley de control NL/Transformada de Park Inversa ==
  f_qs : Inport
  f_ds : Inport  Port=2
  f_0s : Inport  Port=3
  tita_r1 : Inport  Port=4
  MATLAB Function2 : MATLAB Function  TreatAsAtomicUnit=on
  f_as : Outport
  f_bs : Outport  Port=2
  f_cs : Outport  Port=3
  wires:
  tita_r1/1 -> MATLAB Function2/4(tita_r)
  MATLAB Function2/2(f_bs) -> f_bs/1
  MATLAB Function2/1(f_as) -> f_as/1
  f_ds/1 -> MATLAB Function2/2(f_ds)
  MATLAB Function2/3(f_cs) -> f_cs/1
  f_0s/1 -> MATLAB Function2/3(f_0s)
  f_qs/1 -> MATLAB Function2/1(f_qs)

== system Simulacion_con_vd_export/Modelo NL desacoplado con Ley de control NL1/Sistema completo analizado  ==
  v_as : Inport
  v_bs : Inport  Port=2
  v_cs : Inport  Port=3
  T_amb : Inport  Port=4
  T_ld : Inport  Port=5
  g : Inport  Port=6
  Gain : Gain  Gain=P_p
  Subsistema electromecánico : Subsystem
  Subsistema mecánico : Subsystem
  Subsistema térmico1 : Subsystem
  Transformada de Park Directa : Subsystem
  Transformada de Park Inversa : Subsystem
  w_m : Outport
  theta_m : Outport  Port=2
  T_s : Outport  Port=3
  i_as : Outport  Port=4
  i_bs : Outport  Port=5
  i_cs : Outport  Port=6
  Tm : Outport  Port=7
  wires:
  Transformada de Park Inversa/3(f_cs) -> i_cs/1
  Subsistema mecánico/1(w_m) -> w_m/1, Subsistema electromecánico/5(w_m)
  Subsistema electromecánico/3(i_0s) -> Subsistema térmico1/3(i_0s), Transformada de Park Inversa/3(f_0s)
  Transformada de Park Directa/1(fqs) -> Subsistema electromecánico/1(v_qs)
  Subsistema térmico1/2(T_s) -> T_s/1
  Transformada de Park Directa/3(f0s) -> Subsistema electromecánico/3(v_0s)
  Subsistema electromecánico/2(i_ds) -> Subsistema térmico1/2(i_ds), Transformada de Park Inversa/2(f_ds), Subsistema mecánico/2(i_ds)
  Gain/1 -> Transformada de Park Inversa/4(tita_r1), Transformada de Park Directa/4(tita_r)
  T_ld/1 -> Subsistema mecánico/1(T_ld)
  Transformada de Park Directa/2(fds) -> Subsistema electromecánico/2(v_ds)
  Transformada de Park Inversa/2(f_bs) -> i_bs/1
  v_bs/1 -> Transformada de Park Directa/2(fbs)
  T_amb/1 -> Subsistema térmico1/4(T_amb)
  Transformada de Park Inversa/1(f_as) -> i_as/1
  v_as/1 -> Transformada de Park Directa/1(fas)
  Subsistema mecánico/2(theta_m) -> Gain/1, theta_m/1
  v_cs/1 -> Transformada de Park Directa/3(fcs)
  Subsistema electromecánico/1(i_qs) -> Transformada de Park Inversa/1(f_qs), Subsistema mecánico/3(i_qs), Subsistema térmico1/1(i_qs)
  Subsistema térmico1/1(R_s) -> Subsistema electromecánico/4(Rs)
  g/1 -> Subsistema mecánico/4(g)
  Subsistema mecánico/3(Tm) -> Tm/1

== system Simulacion_con_vd_export/Modelo NL desacoplado con Ley de control NL1/Transformada de Park Directa ==
  fas : Inport
  fbs : Inport  Port=2
  fcs : Inport  Port=3
  tita_r : Inport  Port=4
  MATLAB Function1 : MATLAB Function  TreatAsAtomicUnit=on
  fqs : Outport
  fds : Outport  Port=2
  f0s : Outport  Port=3
  wires:
  fas/1 -> MATLAB Function1/1(f_as)
  MATLAB Function1/3(f_0s) -> f0s/1
  MATLAB Function1/2(f_ds) -> fds/1
  fbs/1 -> MATLAB Function1/2(f_bs)
  fcs/1 -> MATLAB Function1/3(f_cs)
  tita_r/1 -> MATLAB Function1/4(tita_r)
  MATLAB Function1/1(f_qs) -> fqs/1

== system Simulacion_con_vd_export/Modelo NL desacoplado con Ley de control NL1/Transformada de Park Inversa ==
  f_qs : Inport
  f_ds : Inport  Port=2
  f_0s : Inport  Port=3
  tita_r1 : Inport  Port=4
  MATLAB Function2 : MATLAB Function  TreatAsAtomicUnit=on
  f_as : Outport
  f_bs : Outport  Port=2
  f_cs : Outport  Port=3
  wires:
  tita_r1/1 -> MATLAB Function2/4(tita_r)
  MATLAB Function2/2(f_bs) -> f_bs/1
  MATLAB Function2/1(f_as) -> f_as/1
  f_ds/1 -> MATLAB Function2/2(f_ds)
  MATLAB Function2/3(f_cs) -> f_cs/1
  f_0s/1 -> MATLAB Function2/3(f_0s)
  f_qs/1 -> MATLAB Function2/1(f_qs)

== system Simulacion_con_vd_export/Modelo NL desacoplado con Ley de control NL2/Sistema completo analizado  ==
  v_as : Inport
  v_bs : Inport  Port=2
  v_cs : Inport  Port=3
  T_amb : Inport  Port=4
  T_ld : Inport  Port=5
  g : Inport  Port=6
  Gain : Gain  Gain=P_p
  Subsistema electromecánico : Subsystem
  Subsistema mecánico : Subsystem
  Subsistema térmico1 : Subsystem
  Transformada de Park Directa : Subsystem
  Transformada de Park Inversa : Subsystem
  w_m : Outport
  theta_m : Outport  Port=2
  T_s : Outport  Port=3
  i_as : Outport  Port=4
  i_bs : Outport  Port=5
  i_cs : Outport  Port=6
  Tm : Outport  Port=7
  wires:
  Transformada de Park Inversa/3(f_cs) -> i_cs/1
  Subsistema mecánico/1(w_m) -> w_m/1, Subsistema electromecánico/5(w_m)
  Subsistema electromecánico/3(i_0s) -> Subsistema térmico1/3(i_0s), Transformada de Park Inversa/3(f_0s)
  Transformada de Park Directa/1(fqs) -> Subsistema electromecánico/1(v_qs)
  Subsistema térmico1/2(T_s) -> T_s/1
  Transformada de Park Directa/3(f0s) -> Subsistema electromecánico/3(v_0s)
  Subsistema electromecánico/2(i_ds) -> Subsistema térmico1/2(i_ds), Transformada de Park Inversa/2(f_ds), Subsistema mecánico/2(i_ds)
  Gain/1 -> Transformada de Park Inversa/4(tita_r1), Transformada de Park Directa/4(tita_r)
  T_ld/1 -> Subsistema mecánico/1(T_ld)
  Transformada de Park Directa/2(fds) -> Subsistema electromecánico/2(v_ds)
  Transformada de Park Inversa/2(f_bs) -> i_bs/1
  v_bs/1 -> Transformada de Park Directa/2(fbs)
  T_amb/1 -> Subsistema térmico1/4(T_amb)
  Transformada de Park Inversa/1(f_as) -> i_as/1
  v_as/1 -> Transformada de Park Directa/1(fas)
  Subsistema mecánico/2(theta_m) -> Gain/1, theta_m/1
  v_cs/1 -> Transformada de Park Directa/3(fcs)
  Subsistema electromecánico/1(i_qs) -> Transformada de Park Inversa/1(f_qs), Subsistema mecánico/3(i_qs), Subsistema térmico1/1(i_qs)
  Subsistema térmico1/1(R_s) -> Subsistema electromecánico/4(Rs)
  g/1 -> Subsistema mecánico/4(g)
  Subsistema mecánico/3(Tm) -> Tm/1

== system Simulacion_con_vd_export/Modelo NL desacoplado con Ley de control NL2/Transformada de Park Directa ==
  fas : Inport
  fbs : Inport  Port=2
  fcs : Inport  Port=3
  tita_r : Inport  Port=4
  MATLAB Function1 : MATLAB Function  TreatAsAtomicUnit=on
  fqs : Outport
  fds : Outport  Port=2
  f0s : Outport  Port=3
  wires:
  fas/1 -> MATLAB Function1/1(f_as)
  MATLAB Function1/3(f_0s) -> f0s/1
  MATLAB Function1/2(f_ds) -> fds/1
  fbs/1 -> MATLAB Function1/2(f_bs)
  fcs/1 -> MATLAB Function1/3(f_cs)
  tita_r/1 -> MATLAB Function1/4(tita_r)
  MATLAB Function1/1(f_qs) -> fqs/1

== system Simulacion_con_vd_export/Modelo NL desacoplado con Ley de control NL2/Transformada de Park Inversa ==
  f_qs : Inport
  f_ds : Inport  Port=2
  f_0s : Inport  Port=3
  tita_r1 : Inport  Port=4
  MATLAB Function2 : MATLAB Function  TreatAsAtomicUnit=on
  f_as : Outport
  f_bs : Outport  Port=2
  f_cs : Outport  Port=3
  wires:
  tita_r1/1 -> MATLAB Function2/4(tita_r)
  MATLAB Function2/2(f_bs) -> f_bs/1
  MATLAB Function2/1(f_as) -> f_as/1
  f_ds/1 -> MATLAB Function2/2(f_ds)
  MATLAB Function2/3(f_cs) -> f_cs/1
  f_0s/1 -> MATLAB Function2/3(f_0s)
  f_qs/1 -> MATLAB Function2/1(f_qs)

== system Simulacion_con_vd_export/Sistema completo LTI/Subsistema electromecánico LTI eq ==
  v_qs : Inport
  Rs : Inport  Port=2
  w_m : Inport  Port=3
  Constant1 : Constant  Value=lambda_m
  Gain6 : Gain  Gain=1/L_q
  Gain7 : Gain  Gain=P_p
  Product5 : Product
  Product6 : Product
  Sum4 : Sum  Inputs=+|-|-
  i_qs(0)=0 : Integrator
  i_qs : Outport
  wires:
  Sum4/1 -> Gain6/1
  Product6/1 -> Sum4/2
  Gain7/1 -> Product6/2
  v_qs/1 -> Sum4/1
  w_m/1 -> Gain7/1
  Constant1/1 -> Product6/1
  i_qs(0)=0/1 -> i_qs/1, Product5/2  "i_qs"
  Product5/1 -> Sum4/3
  Rs/1 -> Product5/1
  Gain6/1 -> i_qs(0)=0/1  "di_qs/dt"

== system Simulacion_con_vd_export/Sistema completo LTI/Subsistema mecánico ==
  T_ld : Inport
  i_ds : Inport  Port=2
  i_qs : Inport  Port=3
  g : Inport  Port=4
  Constant1 : Constant  Value=lambda_m
  Gain10 : Gain  Gain=1/r
  Gain11 : Gain  Gain=1/r
  Gain12 : Gain  Gain=1/J_eq
  Gain13 : Gain  Gain=b_eq
  Gain7 : Gain  Gain=L_d - L_q
  Gain8 : Gain  Gain=3/2 * P_p
  Gain9 : Gain  Gain=k_l
  Product1 : Product
  Product2 : Product
  Sum3 : Sum  Inputs=+|-|-
  Sum4 : Sum  Inputs=|++
  Sum5 : Sum  Inputs=|++
  Trigonometric Function1 : Trigonometry
  theta_m(0)=1 : Integrator
  w_m(0)=1 : Integrator
  w_m : Outport
  theta_m : Outport  Port=2
  Tm : Outport  Port=3
  wires:
  w_m(0)=1/1 -> w_m/1, theta_m(0)=1/1, Gain13/1  "w_m"
  Gain9/1 -> Product2/2
  Gain11/1 -> Trigonometric Function1/1
  i_ds/1 -> Gain7/1
  Constant1/1 -> Sum4/1
  Gain13/1 -> Sum3/3
  Gain10/1 -> Sum3/2
  T_ld/1 -> Sum5/1
  g/1 -> Product2/1
  Trigonometric Function1/1 -> Gain9/1
  theta_m(0)=1/1 -> Gain11/1, theta_m/1  "theta_m"
  Sum5/1 -> Gain10/1
  Product2/1 -> Sum5/2
  Gain8/1 -> Product1/1
  i_qs/1 -> Product1/2
  Sum3/1 -> Gain12/1
  Gain12/1 -> w_m(0)=1/1  "dw_m/dt"
  Sum4/1 -> Gain8/1
  Gain7/1 -> Sum4/2
  Product1/1 -> Sum3/1, Tm/1

== system Simulacion_con_vd_export/Sistema completo LTI/Subsistema térmico LTI eq ==
  i_qs : Inport
  i_ds : Inport  Port=2
  i_0s : Inport  Port=3
  T_amb : Inport  Port=4
  Add : Sum  Inputs=+++
  Gain : Gain  Gain=1/C_ts
  Gain1 : Gain  Gain=R_sREF
  Gain3 : Gain  Gain=1/R_ts_amb
  Gain4 : Gain  Gain=3/2
  Gain5 : Gain  Gain=2
  Math Function : Math  Operator=magnitude^2
  Math Function1 : Math  Operator=magnitude^2
  Math Function2 : Math  Operator=magnitude^2
  Sum1 : Sum  Inputs=|-+
  Sum2 : Sum  Inputs=|-+
  T_s(0) = 40 : Integrator  InitialCondition=40
  T_s : Outport
  wires:
  Math Function2/1 -> Gain5/1
  Math Function/1 -> Add/1
  T_amb/1 -> Sum1/1
  Sum2/1 -> Gain/1
  Sum1/1 -> Gain3/1
  Gain1/1 -> Sum2/2
  i_ds/1 -> Math Function1/1
  Gain/1 -> T_s(0) = 40/1  "dT_s/dt"
  Gain4/1 -> Gain1/1
  T_s(0) = 40/1 -> Sum1/2, T_s/1
  Math Function1/1 -> Add/2
  i_0s/1 -> Math Function2/1
  Add/1 -> Gain4/1
  Gain5/1 -> Add/3
  i_qs/1 -> Math Function/1
  Gain3/1 -> Sum2/1  "dT_s/dt"

== system Simulacion_con_vd_export/Sistema completo LTI/Transformada de Park Inversa ==
  f_qs : Inport
  f_ds : Inport  Port=2
  f_0s : Inport  Port=3
  tita_r1 : Inport  Port=4
  MATLAB Function2 : MATLAB Function  TreatAsAtomicUnit=on
  f_as : Outport
  f_bs : Outport  Port=2
  f_cs : Outport  Port=3
  wires:
  tita_r1/1 -> MATLAB Function2/4(tita_r)
  MATLAB Function2/2(f_bs) -> f_bs/1
  MATLAB Function2/1(f_as) -> f_as/1
  f_ds/1 -> MATLAB Function2/2(f_ds)
  MATLAB Function2/3(f_cs) -> f_cs/1
  f_0s/1 -> MATLAB Function2/3(f_0s)
  f_qs/1 -> MATLAB Function2/1(f_qs)

== system Simulacion_con_vd_export/Sistema completo LTI1/Subsistema electromecánico LTI eq ==
  v_qs : Inport
  Rs : Inport  Port=2
  w_m : Inport  Port=3
  Constant1 : Constant  Value=lambda_m
  Gain6 : Gain  Gain=1/L_q
  Gain7 : Gain  Gain=P_p
  Product5 : Product
  Product6 : Product
  Sum4 : Sum  Inputs=+|-|-
  i_qs(0)=0 : Integrator
  i_qs : Outport
  wires:
  Sum4/1 -> Gain6/1
  Product6/1 -> Sum4/2
  Gain7/1 -> Product6/2
  v_qs/1 -> Sum4/1
  w_m/1 -> Gain7/1
  Constant1/1 -> Product6/1
  i_qs(0)=0/1 -> i_qs/1, Product5/2  "i_qs"
  Product5/1 -> Sum4/3
  Rs/1 -> Product5/1
  Gain6/1 -> i_qs(0)=0/1  "di_qs/dt"

== system Simulacion_con_vd_export/Sistema completo LTI1/Subsistema mecánico ==
  T_ld : Inport
  i_ds : Inport  Port=2
  i_qs : Inport  Port=3
  g : Inport  Port=4
  Constant1 : Constant  Value=lambda_m
  Gain10 : Gain  Gain=1/r
  Gain11 : Gain  Gain=1/r
  Gain12 : Gain  Gain=1/J_eq
  Gain13 : Gain  Gain=b_eq
  Gain7 : Gain  Gain=L_d - L_q
  Gain8 : Gain  Gain=3/2 * P_p
  Gain9 : Gain  Gain=k_l
  Product1 : Product
  Product2 : Product
  Sum3 : Sum  Inputs=+|-|-
  Sum4 : Sum  Inputs=|++
  Sum5 : Sum  Inputs=|++
  Trigonometric Function1 : Trigonometry
  theta_m(0)=1 : Integrator
  w_m(0)=1 : Integrator
  w_m : Outport
  theta_m : Outport  Port=2
  Tm : Outport  Port=3
  wires:
  w_m(0)=1/1 -> w_m/1, theta_m(0)=1/1, Gain13/1  "w_m"
  Gain9/1 -> Product2/2
  Gain11/1 -> Trigonometric Function1/1
  i_ds/1 -> Gain7/1
  Constant1/1 -> Sum4/1
  Gain13/1 -> Sum3/3
  Gain10/1 -> Sum3/2
  T_ld/1 -> Sum5/1
  g/1 -> Product2/1
  Trigonometric Function1/1 -> Gain9/1
  theta_m(0)=1/1 -> Gain11/1, theta_m/1  "theta_m"
  Sum5/1 -> Gain10/1
  Product2/1 -> Sum5/2
  Gain8/1 -> Product1/1
  i_qs/1 -> Product1/2
  Sum3/1 -> Gain12/1
  Gain12/1 -> w_m(0)=1/1  "dw_m/dt"
  Sum4/1 -> Gain8/1
  Gain7/1 -> Sum4/2
  Product1/1 -> Sum3/1, Tm/1

== system Simulacion_con_vd_export/Sistema completo LTI1/Subsistema térmico LTI eq ==
  i_qs : Inport
  i_ds : Inport  Port=2
  i_0s : Inport  Port=3
  T_amb : Inport  Port=4
  Add : Sum  Inputs=+++
  Gain : Gain  Gain=1/C_ts
  Gain1 : Gain  Gain=R_sREF
  Gain3 : Gain  Gain=1/R_ts_amb
  Gain4 : Gain  Gain=3/2
  Gain5 : Gain  Gain=2
  Math Function : Math  Operator=magnitude^2
  Math Function1 : Math  Operator=magnitude^2
  Math Function2 : Math  Operator=magnitude^2
  Sum1 : Sum  Inputs=|-+
  Sum2 : Sum  Inputs=|-+
  T_s(0) = 40 : Integrator  InitialCondition=40
  T_s : Outport
  wires:
  Math Function2/1 -> Gain5/1
  Math Function/1 -> Add/1
  T_amb/1 -> Sum1/1
  Sum2/1 -> Gain/1
  Sum1/1 -> Gain3/1
  Gain1/1 -> Sum2/2
  i_ds/1 -> Math Function1/1
  Gain/1 -> T_s(0) = 40/1  "dT_s/dt"
  Gain4/1 -> Gain1/1
  T_s(0) = 40/1 -> Sum1/2, T_s/1
  Math Function1/1 -> Add/2
  i_0s/1 -> Math Function2/1
  Add/1 -> Gain4/1
  Gain5/1 -> Add/3
  i_qs/1 -> Math Function/1
  Gain3/1 -> Sum2/1  "dT_s/dt"

== system Simulacion_con_vd_export/Sistema completo LTI1/Transformada de Park Inversa ==
  f_qs : Inport
  f_ds : Inport  Port=2
  f_0s : Inport  Port=3
  tita_r1 : Inport  Port=4
  MATLAB Function2 : MATLAB Function  TreatAsAtomicUnit=on
  f_as : Outport
  f_bs : Outport  Port=2
  f_cs : Outport  Port=3
  wires:
  tita_r1/1 -> MATLAB Function2/4(tita_r)
  MATLAB Function2/2(f_bs) -> f_bs/1
  MATLAB Function2/1(f_as) -> f_as/1
  f_ds/1 -> MATLAB Function2/2(f_ds)
  MATLAB Function2/3(f_cs) -> f_cs/1
  f_0s/1 -> MATLAB Function2/3(f_0s)
  f_qs/1 -> MATLAB Function2/1(f_qs)

== system Simulacion_con_vd_export/Sistema completo LTI2/Subsistema electromecánico LTI eq ==
  v_qs : Inport
  Rs : Inport  Port=2
  w_m : Inport  Port=3
  Constant1 : Constant  Value=lambda_m
  Gain6 : Gain  Gain=1/L_q
  Gain7 : Gain  Gain=P_p
  Product5 : Product
  Product6 : Product
  Sum4 : Sum  Inputs=+|-|-
  i_qs(0)=0 : Integrator
  i_qs : Outport
  wires:
  Sum4/1 -> Gain6/1
  Product6/1 -> Sum4/2
  Gain7/1 -> Product6/2
  v_qs/1 -> Sum4/1
  w_m/1 -> Gain7/1
  Constant1/1 -> Product6/1
  i_qs(0)=0/1 -> i_qs/1, Product5/2  "i_qs"
  Product5/1 -> Sum4/3
  Rs/1 -> Product5/1
  Gain6/1 -> i_qs(0)=0/1  "di_qs/dt"

== system Simulacion_con_vd_export/Sistema completo LTI2/Subsistema mecánico ==
  T_ld : Inport
  i_ds : Inport  Port=2
  i_qs : Inport  Port=3
  g : Inport  Port=4
  Constant1 : Constant  Value=lambda_m
  Gain10 : Gain  Gain=1/r
  Gain11 : Gain  Gain=1/r
  Gain12 : Gain  Gain=1/J_eq
  Gain13 : Gain  Gain=b_eq
  Gain7 : Gain  Gain=L_d - L_q
  Gain8 : Gain  Gain=3/2 * P_p
  Gain9 : Gain  Gain=k_l
  Product1 : Product
  Product2 : Product
  Sum3 : Sum  Inputs=+|-|-
  Sum4 : Sum  Inputs=|++
  Sum5 : Sum  Inputs=|++
  Trigonometric Function1 : Trigonometry
  theta_m(0)=1 : Integrator
  w_m(0)=1 : Integrator
  w_m : Outport
  theta_m : Outport  Port=2
  Tm : Outport  Port=3
  wires:
  w_m(0)=1/1 -> w_m/1, theta_m(0)=1/1, Gain13/1  "w_m"
  Gain9/1 -> Product2/2
  Gain11/1 -> Trigonometric Function1/1
  i_ds/1 -> Gain7/1
  Constant1/1 -> Sum4/1
  Gain13/1 -> Sum3/3
  Gain10/1 -> Sum3/2
  T_ld/1 -> Sum5/1
  g/1 -> Product2/1
  Trigonometric Function1/1 -> Gain9/1
  theta_m(0)=1/1 -> Gain11/1, theta_m/1  "theta_m"
  Sum5/1 -> Gain10/1
  Product2/1 -> Sum5/2
  Gain8/1 -> Product1/1
  i_qs/1 -> Product1/2
  Sum3/1 -> Gain12/1
  Gain12/1 -> w_m(0)=1/1  "dw_m/dt"
  Sum4/1 -> Gain8/1
  Gain7/1 -> Sum4/2
  Product1/1 -> Sum3/1, Tm/1

== system Simulacion_con_vd_export/Sistema completo LTI2/Subsistema térmico LTI eq ==
  i_qs : Inport
  i_ds : Inport  Port=2
  i_0s : Inport  Port=3
  T_amb : Inport  Port=4
  Add : Sum  Inputs=+++
  Gain : Gain  Gain=1/C_ts
  Gain1 : Gain  Gain=R_sREF
  Gain3 : Gain  Gain=1/R_ts_amb
  Gain4 : Gain  Gain=3/2
  Gain5 : Gain  Gain=2
  Math Function : Math  Operator=magnitude^2
  Math Function1 : Math  Operator=magnitude^2
  Math Function2 : Math  Operator=magnitude^2
  Sum1 : Sum  Inputs=|-+
  Sum2 : Sum  Inputs=|-+
  T_s(0) = 40 : Integrator  InitialCondition=40
  T_s : Outport
  wires:
  Math Function2/1 -> Gain5/1
  Math Function/1 -> Add/1
  T_amb/1 -> Sum1/1
  Sum2/1 -> Gain/1
  Sum1/1 -> Gain3/1
  Gain1/1 -> Sum2/2
  i_ds/1 -> Math Function1/1
  Gain/1 -> T_s(0) = 40/1  "dT_s/dt"
  Gain4/1 -> Gain1/1
  T_s(0) = 40/1 -> Sum1/2, T_s/1
  Math Function1/1 -> Add/2
  i_0s/1 -> Math Function2/1
  Add/1 -> Gain4/1
  Gain5/1 -> Add/3
  i_qs/1 -> Math Function/1
  Gain3/1 -> Sum2/1  "dT_s/dt"

== system Simulacion_con_vd_export/Sistema completo LTI2/Transformada de Park Inversa ==
  f_qs : Inport
  f_ds : Inport  Port=2
  f_0s : Inport  Port=3
  tita_r1 : Inport  Port=4
  MATLAB Function2 : MATLAB Function  TreatAsAtomicUnit=on
  f_as : Outport
  f_bs : Outport  Port=2
  f_cs : Outport  Port=3
  wires:
  tita_r1/1 -> MATLAB Function2/4(tita_r)
  MATLAB Function2/2(f_bs) -> f_bs/1
  MATLAB Function2/1(f_as) -> f_as/1
  f_ds/1 -> MATLAB Function2/2(f_ds)
  MATLAB Function2/3(f_cs) -> f_cs/1
  f_0s/1 -> MATLAB Function2/3(f_0s)
  f_qs/1 -> MATLAB Function2/1(f_qs)

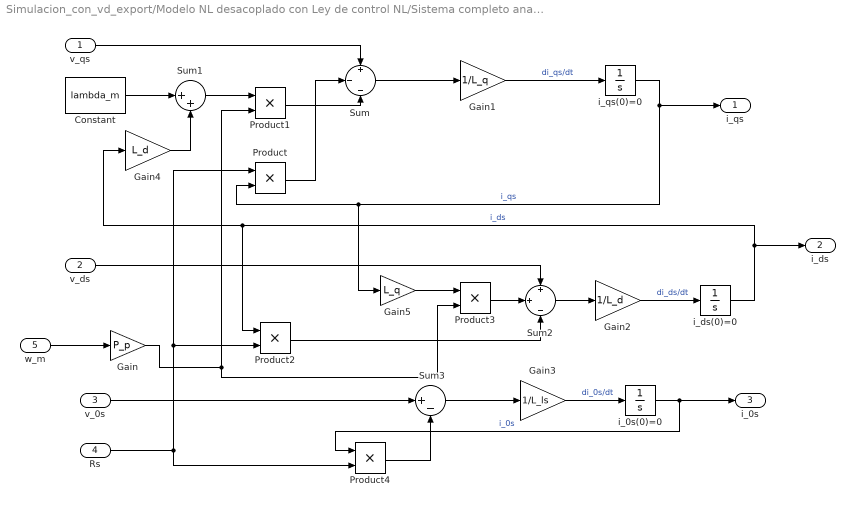
== system Simulacion_con_vd_export/Modelo NL desacoplado con Ley de control NL/Sistema completo analizado /Subsistema electromecánico ==
  v_qs : Inport
  v_ds : Inport  Port=2
  v_0s : Inport  Port=3
  Rs : Inport  Port=4
  w_m : Inport  Port=5
  Constant : Constant  Value=lambda_m
  Gain : Gain  Gain=P_p
  Gain1 : Gain  Gain=1/L_q
  Gain2 : Gain  Gain=1/L_d
  Gain3 : Gain  Gain=1/L_ls
  Gain4 : Gain  Gain=L_d
  Gain5 : Gain  Gain=L_q
  Product{,1..4} (5 alike) : Product
  Sum : Sum  Inputs=+|-|-
  Sum1 : Sum  Inputs=|++
  Sum2 : Sum  Inputs=+|+|-
  Sum3 : Sum  Inputs=|+-
  i_0s(0)=0 : Integrator
  i_ds(0)=0 : Integrator
  i_qs(0)=0 : Integrator
  i_qs : Outport
  i_ds : Outport  Port=2
  i_0s : Outport  Port=3
  wires:
  Gain1/1 -> i_qs(0)=0/1  "di_qs/dt"
  Rs/1 -> Product2/2, Product/1, Product4/2
  i_qs(0)=0/1 -> Gain5/1, Product/2, i_qs/1  "i_qs"
  Sum2/1 -> Gain2/1
  Product1/1 -> Sum/3
  Product4/1 -> Sum3/2
  v_0s/1 -> Sum3/1
  Product3/1 -> Sum2/2
  Gain3/1 -> i_0s(0)=0/1  "di_0s/dt"
  Gain/1 -> Product3/2, Product1/2
  v_qs/1 -> Sum/1
  Sum1/1 -> Product1/1
  Gain5/1 -> Product3/1
  Sum3/1 -> Gain3/1
  i_0s(0)=0/1 -> Product4/1, i_0s/1  "i_0s"
  Product2/1 -> Sum2/3
  Gain2/1 -> i_ds(0)=0/1  "di_ds/dt"
  Constant/1 -> Sum1/1
  Gain4/1 -> Sum1/2
  Sum/1 -> Gain1/1
  Product/1 -> Sum/2
  w_m/1 -> Gain/1
  i_ds(0)=0/1 -> Product2/1, Gain4/1, i_ds/1  "i_ds"
  v_ds/1 -> Sum2/1
